simulink model "QR2Dsim"  (R2013b)
settings: Solver=ode3  StartTime=0.0  StopTime=Tend_sim  FixedStep=.01  RelTol=1e-3
values from neighbouring files (symbols this model uses):
  b = 0.1    [QR2Drunfile.m]
  ctauf = 8.004e-3    (= 0.008004)    [QR2Drunfile.m]
  d = 0.1    [QR2Drunfile.m]
  DeltaR = [0.2; -0.1; 0.02]    [QR2Drunfile.m]
  Deltax = [-0.5; 0.2; 1]    [QR2Drunfile.m]
  dxL0 = 0    [QR2Drunfile.m]
  dyL0 = 0    [QR2Drunfile.m]
  dzL0 = 0    [QR2Drunfile.m]
  e3 = [0;0;1]    [QR2Drunfile.m]
  fc = (mQ+mL)*g    (= 44.5374)    [QR2Drunfile.m]
  fsat = [-1000 1000]    [QR2Drunfile.m]
  g = 9.81    [QR2Drunfile.m]
  I = diag([Ixx Iyy Izz])    [QR2Drunfile.m]
  Ir = 0.5    [QR2Drunfile.m]
  Ixx = 0.0820    (= 0.082)    [QR2Drunfile.m]
  Iyy = 0    [QR2Drunfile.m]
  Izz = 0    [QR2Drunfile.m]
  kdL = 1.4    [QR2Drunfile.m]
  kdQ = 5.6*mQ*.75    (= 18.228)    [QR2Drunfile.m]
  kdxL = 1    [QR2Drunfile.m]
  kOmega = kOmega_phi*eye(3)    [QR2Drunfile.m]
  kpL = 1.2    [QR2Drunfile.m]
  kpQ = 16*mQ    (= 69.44)    [QR2Drunfile.m]
  kpxL = 5    [QR2Drunfile.m]
  kR = kR_phi*eye(3)    [QR2Drunfile.m]
  l = 0.315    [QR2Drunfile.m]
  lL = 0.4    [QR2Drunfile.m]
  mL = 0.2    [QR2Drunfile.m]
  mode = 2    [QR2Drunfile.m]
  mQ = 4.34    [QR2Drunfile.m]
  omega0 = [0;0;0]    [QR2Drunfile.m]
  phiL0 = deg2rad(190)    [QR2Drunfile.m]
  phiLd = 0    [QR2Drunfile.m]
  phiQ0 = deg2rad(0)    [QR2Drunfile.m]
  phiQd = 0    [QR2Drunfile.m]
  pL0 = 0    [QR2Drunfile.m]
  pQ0 = 0    [QR2Drunfile.m]
  psiL0 = 0    [QR2Drunfile.m]
  psiQ0 = 0    [QR2Drunfile.m]
  qL0 = 0    [QR2Drunfile.m]
  qQ0 = 0    [QR2Drunfile.m]
  qvec0 = [0; sin(phiL0); cos(phiL0)]    [QR2Drunfile.m]
  Rinit = Rx    [QR2Drunfile.m]
  rL0 = 0    [QR2Drunfile.m]
  rQ0 = 0    [QR2Drunfile.m]
  thetaL0 = 0    [QR2Drunfile.m]
  thetaQ0 = 0    [QR2Drunfile.m]
  xLd = [0; 0; 0]    [QR2Drunfile.m]
undefined symbols (not defined in the file or in its folder): dx0, dy0, dz0, kv, kx, m, p0, q0, r0, x0, y0, z0
libraries: simulink_extras x10, vrlib x9, dspmathops x2
(part 2 of 2)

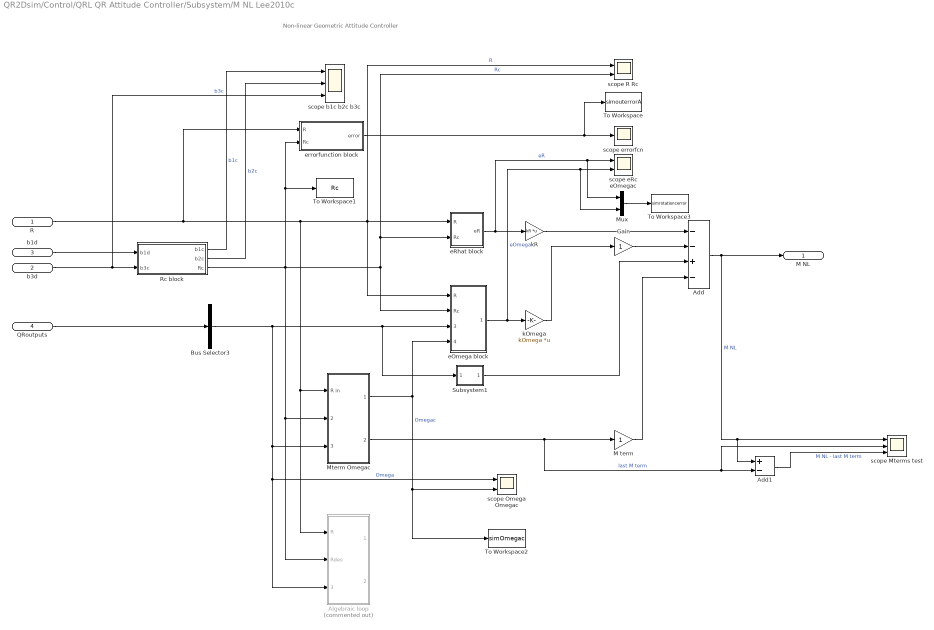
== system QR2Dsim/Control/QRL QR Attitude Controller/Subsystem/M NL Lee2010c ==
  note: Non-linear Geometric Attitude Controller
  R : Inport
  b3d : Inport  Port=2
  b1d : Inport  Port=3
  QRoutputs : Inport  Port=4
  Add : Sum  Inputs=--+-
  Add1 : Sum  Inputs=+-
  Algebraic loop : Subsystem  Commented=on
  Bus Selector3 : BusSelector  OutputSignals=OmegaL  OutputAsBus=on
  Gain : Gain
  M term : Gain
  Mterm Omegac : Subsystem
  Mux : Mux  Inputs=2
  Rc block : MATLAB Function  TreatAsAtomicUnit=on
  Subsystem1 : Subsystem
      mask Display: disp('\Omega \times I\Omega','texmode','on')
  To Workspace : ToWorkspace  VariableName=simouterrorA  SampleTime=-1  SaveFormat=Structure With Time
  To Workspace1 : ToWorkspace  VariableName=Rc  SampleTime=-1  SaveFormat=Structure With Time
  To Workspace2 : ToWorkspace  VariableName=simOmegac  SampleTime=-1  SaveFormat=Structure With Time
  To Workspace3 : ToWorkspace  VariableName=simrotationcerror  SampleTime=-1  SaveFormat=Structure With Time
  eOmega block : MATLAB Function  TreatAsAtomicUnit=on
  eRhat block : MATLAB Function  TreatAsAtomicUnit=on
  errorfunction block : MATLAB Function  TreatAsAtomicUnit=on
  kOmega : Gain  Gain=kOmega  Multiplication=Matrix(K*u)
  kR : Gain  Gain=kR  Multiplication=Matrix(K*u)
  scope Mterms test : Scope  NumInputPorts=3
      settings: YMin=-5~-5~-5  YMax=5~5~5  SaveName=ScopeData13
  scope Omega Omegac : Scope  NumInputPorts=2
      settings: ShowLegends=on  YMin=-5~-5  YMax=5~5  SaveName=scopeOmegac
  scope R Rc : Scope  NumInputPorts=2
      settings: ShowLegends=on  YMin=-5~-5  YMax=5~5  SaveName=ScopeData11
  scope b1c b2c b3c : Scope  NumInputPorts=3
      settings: ShowLegends=on  YMin=-5~-5~-5  YMax=5~5~5  SaveName=ScopeData10
  scope eRc eOmegac : Scope  NumInputPorts=2
      settings: YMin=-5~-5  YMax=5~5  SaveName=ScopeData8
  scope errorfcn : Scope
      settings: SaveName=scopeerrorfnc
  M NL : Outport
  wires:
  R/1 -> eOmega block/1(R), scope R Rc/1, eRhat block/1(R), Algebraic loop/1(R), Mterm Omegac/1(R in), errorfunction block/1(R)  "R"
  kR/1 -> Add/1
  kOmega/1 -> Gain/1
  QRoutputs/1 -> Bus Selector3/1
  Bus Selector3/1 -> eOmega block/3(Omega), Subsystem1/1(Omega), Algebraic loop/3(Omega), scope Omega Omegac/1, Mterm Omegac/3(Omega in)  "Omega"
  Rc block/3(Rc) -> errorfunction block/2(Rc), To Workspace1/1, eOmega block/2(Rc), scope R Rc/2, eRhat block/2(Rc), Algebraic loop/2(Rdes), Mterm Omegac/2(Rdes in)  "Rc"
  Subsystem1/1(Out1) -> Add/3
  Add/1 -> Add1/1, scope Mterms test/1, M NL/1  "M NL"
  errorfunction block/1(error) -> To Workspace/1, scope errorfcn/1
  Mterm Omegac/2(M term) -> M term/1, scope Mterms test/2, Add1/2  "last M term"
  Mterm Omegac/1(Omegades) -> To Workspace2/1, scope Omega Omegac/2, eOmega block/4(Omegac)  "Omegac"
  Gain/1 -> Add/2
  M term/1 -> Add/4
  Add1/1 -> scope Mterms test/3  "M NL - last M term"
  b3d/1 -> scope b1c b2c b3c/3, Rc block/2(b3c)  "b3c"
  b1d/1 -> Rc block/1(b1d)
  Rc block/2(b2c) -> scope b1c b2c b3c/2  "b2c"
  Rc block/1(b1c) -> scope b1c b2c b3c/1  "b1c"
  eRhat block/1(eR) -> Mux/1, scope eRc eOmegac/1, kR/1  "eR"
  eOmega block/1(eOmega) -> Mux/2, scope eRc eOmegac/2, kOmega/1  "eOmega"
  Mux/1 -> To Workspace3/1

== system QR2Dsim/Control/QRL QR Attitude Controller/Subsystem/M lin ==
  note: Linear Attitude Controller
  QRoutputs : Inport
  Add : Sum  Inputs=--
  Bus Selector3 : BusSelector  OutputSignals=OmegaL
  Constant : Constant  Value=[0;0;0]
  eR lin block : MATLAB Function  TreatAsAtomicUnit=on
  kOmega : Gain  Gain=kOmega  Multiplication=Matrix(K*u)
  kR : Gain  Gain=kR  Multiplication=Matrix(K*u)
  M lin : Outport
  wires:
  QRoutputs/1 -> Bus Selector3/1
  Bus Selector3/1 -> kOmega/1  "<OmegaL>"
  eR lin block/1(eRlin) -> kR/1  "eR lin"
  kR/1 -> Add/1
  kOmega/1 -> Add/2
  Add/1 -> M lin/1  "M lin"
  Constant/1 -> eR lin block/2(angles), eR lin block/1(anglesdes)  "anglesdes"

== system QR2Dsim/Control/QRL QR Attitude Controller/Subsystem1/Mterm Omegad ==
  R in : Inport
  Rdes in : Inport  Port=2
  Omega in : Inport  Port=3
  Derivative : Derivative  CoefficientInTFapproximation=c_der
  Gain : Gain
  Gain1 : Gain
  I : Gain  Gain=I  Multiplication=Matrix(K*u)
  Omegac block : MATLAB Function  TreatAsAtomicUnit=on
  Subsystem : Subsystem
  Sum : Sum  Inputs=|+-
  scope Omega Omegad : Scope  NumInputPorts=2
      settings: ShowLegends=on  YMin=-5~-5  YMax=5~5  SaveName=ScopeData22
  Omegades : Outport
  M term : Outport  Port=2
  wires:
  Omegac block/1(Omegad) -> scope Omega Omegad/2, Omegades/1, Subsystem/4(Omegad)  "Omegad"
  Rdes in/1 -> Derivative/1, Omegac block/1(Rd), Subsystem/2(Rd)
  R in/1 -> Subsystem/1(R)
  Omega in/1 -> scope Omega Omegad/1, Subsystem/3(Omega)
  Subsystem/1(Out1) -> Gain1/1
  Sum/1 -> I/1
  Gain/1 -> Sum/2
  Subsystem/2(Out2) -> Gain/1
  I/1 -> M term/1  "M term"
  Gain1/1 -> Sum/1
  Derivative/1 -> Omegac block/2(dRd)  "dRdesTR"

== system QR2Dsim/Control/QRL QR Attitude Controller/Subsystem1/Subsystem1 ==
  Omega : Inport
  Cross Product : vrlib/Utilities/Cross Product
  I : Gain  Gain=I  Multiplication=Matrix(K*u)
  Product1 : Product  Multiplication=Matrix(*)
  Terminator : Terminator
  fcnhat : MATLAB Function  TreatAsAtomicUnit=on
  Out1 : Outport
  wires:
  Omega/1 -> Cross Product/1, I/1, fcnhat/1(A)
  fcnhat/1(fcnhat) -> Product1/1
  I/1 -> Cross Product/2, Product1/2
  Cross Product/1 -> Out1/1
  Product1/1 -> Terminator/1

== system QR2Dsim/Control/QRL QR Attitude Controller/Subsystem/M NL Lee2010/Mterm Omegad ==
  R in : Inport
  Rdes in : Inport  Port=2
  Omega in : Inport  Port=3
  Derivative : Derivative  CoefficientInTFapproximation=c_der
  Gain : Gain
  Gain1 : Gain
  I : Gain  Gain=I  Multiplication=Matrix(K*u)
  Omegac block : MATLAB Function  TreatAsAtomicUnit=on
  Subsystem : Subsystem
  Sum : Sum  Inputs=|+-
  scope Omega Omegad : Scope  NumInputPorts=2
      settings: ShowLegends=on  YMin=-5~-5  YMax=5~5  SaveName=ScopeData22
  Omegades : Outport
  M term : Outport  Port=2
  wires:
  Omegac block/1(Omegad) -> scope Omega Omegad/2, Omegades/1, Subsystem/4(Omegad)  "Omegad"
  Rdes in/1 -> Derivative/1, Omegac block/1(Rd), Subsystem/2(Rd)
  R in/1 -> Subsystem/1(R)
  Omega in/1 -> scope Omega Omegad/1, Subsystem/3(Omega)
  Subsystem/1(Out1) -> Gain1/1
  Sum/1 -> I/1
  Gain/1 -> Sum/2
  Subsystem/2(Out2) -> Gain/1
  I/1 -> M term/1  "M term"
  Gain1/1 -> Sum/1
  Derivative/1 -> Omegac block/2(dRd)  "dRdesTR"

== system QR2Dsim/Control/QRL QR Attitude Controller/Subsystem/M NL Lee2010/Subsystem1 ==
  Omega : Inport
  Cross Product : vrlib/Utilities/Cross Product
  I : Gain  Gain=I  Multiplication=Matrix(K*u)
  Product1 : Product  Multiplication=Matrix(*)
  Terminator : Terminator
  fcnhat : MATLAB Function  TreatAsAtomicUnit=on
  Out1 : Outport
  wires:
  Omega/1 -> Cross Product/1, I/1, fcnhat/1(A)
  fcnhat/1(fcnhat) -> Product1/1
  I/1 -> Cross Product/2, Product1/2
  Cross Product/1 -> Out1/1
  Product1/1 -> Terminator/1

== system QR2Dsim/Control/QRL QR Attitude Controller/Subsystem/M NL Lee2010c/Algebraic loop ==
  R : Inport
  Rdes : Inport  Port=2
  Omega : Inport  Port=3
  Derivative1 : Derivative
  I : Gain  Gain=I  Multiplication=Matrix(K*u)
  I1 : Gain
  M term block : MATLAB Function  TreatAsAtomicUnit=on
  R block : Subsystem
      mask Display: disp('R_{d}^TR\prime_{d} = \Omega_{d,\times}','texmode','on')
  Scope Omegades : Scope  NumInputPorts=2
      settings: ShowLegends=on  YMin=-5~-5  YMax=5~5
  Scope fcnhat : Scope  NumInputPorts=2
      settings: ShowLegends=on  YMin=-5~-5  YMax=5~5  SaveName=ScopeData2
  Sum : Sum  Inputs=|+-
  M term : Outport
  Omegades : Outport  Port=2
  wires:
  Omega/1 -> M term block/3(Omega), Scope fcnhat/1  "Omega"
  Derivative1/1 -> Scope Omegades/2, M term block/5(dOmegades)  "dOmegades"
  I/1 -> M term/1
  R block/1(Omegades) -> Derivative1/1, Omegades/1, Scope fcnhat/2, Scope Omegades/1, M term block/4(Omegades)  "Omegades"
  R/1 -> M term block/1(R)
  Rdes/1 -> M term block/2(Rdes), R block/1(Rdes in)
  M term block/1(Out1) -> Sum/1
  M term block/2(Out2) -> I1/1
  Sum/1 -> I/1
  I1/1 -> Sum/2

== system QR2Dsim/Control/QRL QR Attitude Controller/Subsystem/M NL Lee2010c/Mterm Omegac ==
  R in : Inport
  Rdes in : Inport  Port=2
  Omega in : Inport  Port=3
  Derivative : Derivative  CoefficientInTFapproximation=c_der
  Gain : Gain
  Gain1 : Gain
  I : Gain  Gain=I  Multiplication=Matrix(K*u)
  Omegac block : MATLAB Function  TreatAsAtomicUnit=on
  Subsystem : Subsystem
  Sum : Sum  Inputs=|+-
  scope Omega Omegac : Scope  NumInputPorts=2
      settings: ShowLegends=on  YMin=-5~-5  YMax=5~5  SaveName=ScopeData22
  Omegades : Outport
  M term : Outport  Port=2
  wires:
  Rdes in/1 -> Subsystem/2(Rc), Omegac block/1(Rc), Derivative/1  "Rc"
  R in/1 -> Subsystem/1(R)  "R"
  Omega in/1 -> scope Omega Omegac/1, Subsystem/3(Omega)  "Omega"
  Subsystem/1(Out1) -> Gain1/1
  Sum/1 -> I/1
  Gain/1 -> Sum/2
  Subsystem/2(Out2) -> Gain/1
  I/1 -> M term/1  "M term"
  Gain1/1 -> Sum/1
  Omegac block/1(Omegac) -> Subsystem/4(Omegac), scope Omega Omegac/2, Omegades/1  "Omegac"
  Derivative/1 -> Omegac block/2(dRc)  "dRc"

== system QR2Dsim/Control/QRL QR Attitude Controller/Subsystem/M NL Lee2010c/Subsystem1 ==
  Omega : Inport
  Cross Product : vrlib/Utilities/Cross Product
  I : Gain  Gain=I  Multiplication=Matrix(K*u)
  Product1 : Product  Multiplication=Matrix(*)
  Terminator : Terminator
  fcnhat : MATLAB Function  TreatAsAtomicUnit=on
  Out1 : Outport
  wires:
  Omega/1 -> Cross Product/1, I/1, fcnhat/1(A)
  fcnhat/1(fcnhat) -> Product1/1
  I/1 -> Cross Product/2, Product1/2
  Cross Product/1 -> Out1/1
  Product1/1 -> Terminator/1

== system QR2Dsim/Control/QRL QR Attitude Controller/Subsystem1/Mterm Omegad/Subsystem ==
  R : Inport
  Rd : Inport  Port=2
  Omega : Inport  Port=3
  Omegad : Inport  Port=4
  Derivative1 : Derivative
  M term block : MATLAB Function  TreatAsAtomicUnit=on
  Scope Mterms : Scope  NumInputPorts=2
      settings: ShowLegends=on  YMin=-5~-5  YMax=5~5  SaveName=ScopeData23
  Scope Omega Omegad : Scope  NumInputPorts=2
      settings: ShowLegends=on  YMin=-5~-5  YMax=5~5  SaveName=ScopeData2
  Scope Omegad dOmegad : Scope  NumInputPorts=2
      settings: ShowLegends=on  YMin=-5~-5  YMax=5~5
  Scope R Rd : Scope  NumInputPorts=3
      settings: ShowLegends=on  YMin=-5~-5~-5  YMax=5~5~5  SaveName=ScopeData24
  Out1 : Outport
  Out2 : Outport  Port=2
  wires:
  Omega/1 -> M term block/3(Omega), Scope Omega Omegad/1  "Omega"
  Derivative1/1 -> Scope Omegad dOmegad/2, M term block/5(dOmegad)  "dOmegad"
  M term block/1(Out1) -> Scope Mterms/1, Out1/1
  Omegad/1 -> Derivative1/1, Scope Omega Omegad/2, Scope Omegad dOmegad/1, M term block/4(Omegad)  "Omegad"
  R/1 -> Scope R Rd/1, M term block/1(R)
  Rd/1 -> Scope R Rd/2, M term block/2(Rd)  "Rd"
  M term block/2(Out2) -> Scope Mterms/2, Out2/1
  M term block/3(Out3) -> Scope R Rd/3

== system QR2Dsim/Control/QRL QR Attitude Controller/Subsystem/M NL Lee2010/Mterm Omegad/Subsystem ==
  R : Inport
  Rd : Inport  Port=2
  Omega : Inport  Port=3
  Omegad : Inport  Port=4
  Derivative1 : Derivative
  M term block : MATLAB Function  TreatAsAtomicUnit=on
  Scope Mterms : Scope  NumInputPorts=2
      settings: ShowLegends=on  YMin=-5~-5  YMax=5~5  SaveName=ScopeData23
  Scope Omega Omegad : Scope  NumInputPorts=2
      settings: ShowLegends=on  YMin=-5~-5  YMax=5~5  SaveName=ScopeData2
  Scope Omegad dOmegad : Scope  NumInputPorts=2
      settings: ShowLegends=on  YMin=-5~-5  YMax=5~5
  Scope R Rd : Scope  NumInputPorts=3
      settings: ShowLegends=on  YMin=-5~-5~-5  YMax=5~5~5  SaveName=ScopeData24
  Out1 : Outport
  Out2 : Outport  Port=2
  wires:
  Omega/1 -> M term block/3(Omega), Scope Omega Omegad/1  "Omega"
  Derivative1/1 -> Scope Omegad dOmegad/2, M term block/5(dOmegad)  "dOmegad"
  M term block/1(Out1) -> Scope Mterms/1, Out1/1
  Omegad/1 -> Derivative1/1, Scope Omega Omegad/2, Scope Omegad dOmegad/1, M term block/4(Omegad)  "Omegad"
  R/1 -> Scope R Rd/1, M term block/1(R)
  Rd/1 -> Scope R Rd/2, M term block/2(Rd)  "Rd"
  M term block/2(Out2) -> Scope Mterms/2, Out2/1
  M term block/3(Out3) -> Scope R Rd/3

== system QR2Dsim/Control/QRL QR Attitude Controller/Subsystem/M NL Lee2010c/Algebraic loop/R block ==
  Rdes in : Inport
  Integrator : Integrator  InitialConditionSource=external  ContinuousStateAttributes='R'
  Math Function : Math  Operator=transpose  SaturateOnIntegerOverflow=on
  Product : Product  Inputs=**  Multiplication=Matrix(*)
  Product1 : Product  Inputs=**  Multiplication=Matrix(*)
  v block : MATLAB Function  TreatAsAtomicUnit=on
  Omegades : Outport
  wires:
  Rdes in/1 -> Integrator/2
  Integrator/1 -> Product/1, Math Function/1
  Math Function/1 -> Product1/1
  Product/1 -> Product1/2, Integrator/1
  Product1/1 -> v block/1(hat), Product/2
  v block/1(vec) -> Omegades/1

== system QR2Dsim/Control/QRL QR Attitude Controller/Subsystem/M NL Lee2010c/Mterm Omegac/Subsystem ==
  R : Inport
  Rc : Inport  Port=2
  Omega : Inport  Port=3
  Omegac : Inport  Port=4
  Derivative1 : Derivative
  M term block : MATLAB Function  TreatAsAtomicUnit=on
  Scope Mterms : Scope  NumInputPorts=2
      settings: ShowLegends=on  YMin=-5~-5  YMax=5~5  SaveName=ScopeData23
  Scope Omega Omegac : Scope  NumInputPorts=2
      settings: ShowLegends=on  YMin=-5~-5  YMax=5~5  SaveName=ScopeData2
  Scope Omegac dOmegac : Scope  NumInputPorts=2
      settings: ShowLegends=on  YMin=-5~-5  YMax=5~5
  Scope R Rdes : Scope  NumInputPorts=3
      settings: ShowLegends=on  YMin=-5~-5~-5  YMax=5~5~5  SaveName=ScopeData24
  Out1 : Outport
  Out2 : Outport  Port=2
  wires:
  Omega/1 -> M term block/3(Omega), Scope Omega Omegac/1  "Omega"
  Derivative1/1 -> Scope Omegac dOmegac/2, M term block/5(dOmegac)  "dOmegac"
  M term block/1(Out1) -> Scope Mterms/1, Out1/1
  Omegac/1 -> Derivative1/1, Scope Omega Omegac/2, Scope Omegac dOmegac/1, M term block/4(Omegac)  "Omegac"
  R/1 -> Scope R Rdes/1, M term block/1(R)  "R"
  Rc/1 -> Scope R Rdes/2, M term block/2(Rc)  "Rc"
  M term block/2(Out2) -> Out2/1, Scope Mterms/2
  M term block/3(Out3) -> Scope R Rdes/3

== matlab function QR2Dsim/QR Subsystem/omegarot block/fcnomega ==
  data: var input; M input size=3; f input; omegai output size=4
function omegai = fcn(var,M,f)
%omega = [omega_1^2;omega_2^2;omega_3^2;omega_4^2]

b = var(1);
d = var(2);
l = var(3);

%check if Gamma is invertible?
Gamma = [b b b b;0 -l*b 0 l*b;l*b 0 -l*b 0;-d d -d d];

QRinput = [f;M];

omegai = Gamma\QRinput;

== matlab function QR2Dsim/QR Subsystem/fi block/fcnf ==
  data: var input; M input size=3; f input; fi output size=4
function fi = fcn(var,M, f)
%omega = [omega_1^2;omega_2^2;omega_3^2;omega_4^2]

l = var(1);
ctauf = var(2);

%check if Gamma is invertible?
Gamma = [1 1 1 1;0 -l 0 l;l 0 -l 0;-ctauf ctauf -ctauf ctauf];

QRinput = [f;M];

fi = Gamma\QRinput;

== matlab function QR2Dsim/QR Subsystem/R block/MATLAB Function1 ==
  data: R input size=[3 3]; RR output size=[3 3]
function RR = fcn(R)
%#codegen
RR = R*R.';

== matlab function QR2Dsim/QR Subsystem/dOmega block/Subsystem2/fcnhat1 ==
  data: A input; fcnhat output
function fcnhat = fcn(A)

a = A(1);
b = A(2);
c = A(3);
fcnhat = [0 -c b; 
          c 0 -a;
         -b a 0];

== matlab function QR2Dsim/Control/QRL QR Attitude Controller/Subsystem1/Mterm Omegad/Omegac block ==
  data: Rd input size=[3 3]; dRd input size=[3 3]; Omegad output size=3
function Omegad = fcnOmegad(Rd,dRd)

Omegadhat = Rd.'*dRd;
Omegad = [Omegadhat(6);-Omegadhat(3);Omegadhat(2)];

== matlab function QR2Dsim/QR Subsystem/dOmega block/Subsystem2/fcnomega ==
  data: omega input; fcnomega output
function fcnomega = fcn(omega)

fcnomega = omega(2)+omega(4)-omega(1)-omega(3);

== matlab function QR2Dsim/QR-Load Subsystem/R block/dR block ==
  data: R input size=[3 3]; dR output size=[3 3]; Omega input size=3
function dR = fcn(R,Omega)
%#codegen
p = Omega(1);
q = Omega(2);
r = Omega(3);

Omegahat = [0 -r  q;
            r  0 -p;
           -q  p  0];

dR = R*Omegahat;
% R1 = R;

== matlab function QR2Dsim/Control/QRL QR Attitude Controller/Subsystem/M NL Lee2010/eRhat block ==
  data: R input size=[3 3]; Rdes input size=[3 3]; eR output size=3
function eR = fcnR(R,Rdes)
% Z-X-Y psi-phi-theta

eRhat = (Rdes.'*R-R.'*Rdes);

eR = 0.5*[eRhat(6);-eRhat(3);eRhat(2)];

== matlab function QR2Dsim/QR-Load Subsystem/dOmegaQ block/Subsystem1/fcnhat ==
  data: A input size=[3 1]; fcnhat output size=[3 3]
function fcnhat = fcn(A)

a = A(1);
b = A(2);
c = A(3);
fcnhat = [0 -c b; 
          c 0 -a;
         -b a 0];

== matlab function QR2Dsim/Control/QRL QR Attitude Controller/Subsystem/M lin/eR lin block ==
  data: anglesdes input size=[3 1]; angles input size=[3 1]; eRlin output size=3
function eRlin = fcnR(anglesdes,angles)
% Z-X-Y psi-phi-theta
% Rdes =  R(psi0+dpsi, dphi, dtheta)
% R = R(psi0,0,0)

% dphi   = anglesdes(1) - angles(1);
% dtheta = anglesdes(2) - angles(2);
% dpsi   = anglesdes(3) - angles(3);

dphi   = angles(1);
dtheta = angles(2);
dpsi   = angles(3);

eRlin  = [dphi; dtheta; dpsi];
% Of toch: 
% eRlin  = [-dphi; -dtheta; -dpsi];

== matlab function QR2Dsim/Control/QRL QR Attitude Controller/Subsystem/M NL Lee2010/eOmega block ==
  data: R input size=[3 3]; Rd input size=[3 3]; eOmega output size=3; Omega input size=[3 1]; Omegad input size=[3 1]
function eOmega = fcnR(R,Rd,Omega,Omegad)
% Z-X-Y psi-phi-theta

eOmega = Omega - R.'*Rd*Omegad;

== matlab function QR2Dsim/Control/QRL QR Attitude Controller/Subsystem/M NL Lee2010/Rdes block ==
  data: b2d output; b1d input size=[3 1]; Rdes output size=[3 3]; b3d input size=[3 1]
function [b2d,Rdes] = fcnRdes(b1d,b3d)
%
b2d = cross(b3d,b1d);
Rdes = [b1d b2d b3d];

== matlab function QR2Dsim/QR-Load Subsystem/dOmegaQ block/Subsystem2/fcnhat1 ==
  data: A input; fcnhat output
function fcnhat = fcn(A)

a = A(1);
b = A(2);
c = A(3);
fcnhat = [0 -c b; 
          c 0 -a;
         -b a 0];

== matlab function QR2Dsim/Control/QRL QR Attitude Controller/Subsystem/M NL Lee2010/Subsystem1/fcnhat ==
  data: A input size=[3 1]; fcnhat output size=[3 3]
function fcnhat = fcn(A)

a = A(1);
b = A(2);
c = A(3);
fcnhat = [0 -c b; 
          c 0 -a;
         -b a 0];

== matlab function QR2Dsim/QR-Load Subsystem/dOmegaQ block/Subsystem2/fcnomega ==
  data: omega input; fcnomega output
function fcnomega = fcn(omega)

fcnomega = omega(2)+omega(4)-omega(1)-omega(3);

== matlab function QR2Dsim/QR Subsystem/R block/dR block ==
  data: R input size=[3 3]; dR output size=[3 3]; Omega input size=3
function dR = fcn(R,Omega)
%#codegen
p = Omega(1);
q = Omega(2);
r = Omega(3);

Omegahat = [0 -r  q;
            r  0 -p;
           -q  p  0];

dR = R*Omegahat;
% R1 = R;

== matlab function QR2Dsim/Control/QRL QR Attitude Controller/Subsystem/M NL Lee2010/errorfunction block ==
  data: R input size=[3 3]; Rdes input size=[3 3]; error output
function error = fcn(R,Rdes)

error = 0.5*trace(eye(3)-Rdes.'*R);

== matlab function QR2Dsim/QR Subsystem/dOmega block/Subsystem1/fcnhat ==
  data: A input size=[3 1]; fcnhat output size=[3 3]
function fcnhat = fcn(A)

a = A(1);
b = A(2);
c = A(3);
fcnhat = [0 -c b; 
          c 0 -a;
         -b a 0];

== matlab function QR2Dsim/Control/QRL QR Attitude Controller/Subsystem/M NL Lee2010c/Algebraic loop/M term block ==
  data: R input size=[3 3]; Rdes input size=[3 3]; Out1 output size=3; Omega input size=3; Omegades input size=3; dOmegades input; Out2 output
function [Out1,Out2] = fcnR(R,Rdes,Omega,Omegades,dOmegades)
% Z-X-Y psi-phi-theta

p = Omega(1);
q = Omega(2);
r = Omega(3);

Omegahat = [0 -r  q;
            r  0 -p;
           -q  p  0];

Out1 = Omegahat*R.'*Rdes*Omegades;
Out2 = R.'*Rdes*dOmegades;

== matlab function QR2Dsim/Control/QRL QR Attitude Controller/Subsystem/M NL Lee2010/Mterm Omegad/Subsystem/M term block ==
  data: R input size=[3 3]; Rd input size=[3 3]; Out1 output size=3; Omega input size=3; Omegad input size=3; dOmegad input; Out2 output; Out3 output
function [Out1,Out2,Out3] = fcnR(R,Rd,Omega,Omegad,dOmegad)
% Z-X-Y psi-phi-theta

p = Omega(1);
q = Omega(2);
r = Omega(3);

Omegahat = [0 -r  q;
            r  0 -p;
           -q  p  0];

Out1 = Omegahat*R.'*Rd*Omegad;
Out2 = R.'*Rd*dOmegad;
Out3 = R.'*Rd;

== matlab function QR2Dsim/Control/QRL QR Attitude Controller/Subsystem/M NL Lee2010c/Algebraic loop/R block/v block ==
  data: hat input size=[3 3]; vec output size=3
function vec = fcn(hat)

vec = [hat(6); -hat(3); hat(2)];

== matlab function QR2Dsim/Control/QRL QR Attitude Controller/Subsystem/M NL Lee2010c/Rc block ==
  data: b1c output; b2c output; b1d input size=[3 1]; Rc output size=[3 3]; b3c input size=[3 1]
function [b1c,b2c,Rc] = fcnRc(b1d,b3c)
%
b1c = -cross(b3c,(cross(b3c,b1d)/norm(cross(b3c,b1d))));
% b1c = -cross(b3c,normc(cross(b3c,b1d)));
b2c = cross(b3c,b1c);
Rc = [b1c b2c b3c];
% Rc = Rc.';

== matlab function QR2Dsim/Control/QRL QR Attitude Controller/Subsystem/M NL Lee2010c/Mterm Omegac/Omegac block ==
  data: Rc input size=[3 3]; dRc input size=[3 3]; Omegac output size=3
function Omegac = fcnOmegac(Rc,dRc)

Omegachat = Rc.'*dRc;
Omegac = [Omegachat(6);-Omegachat(3);Omegachat(2)];

== matlab function QR2Dsim/Control/QRL QR Attitude Controller/Subsystem/M NL Lee2010c/Mterm Omegac/Subsystem/M term block ==
  data: R input size=[3 3]; Rc input size=[3 3]; Out1 output size=3; Omega input size=3; Omegac input size=3; dOmegac input; Out2 output; Out3 output
function [Out1,Out2,Out3] = fcnMterm(R,Rc,Omega,Omegac,dOmegac)
% Z-X-Y psi-phi-theta

p = Omega(1);
q = Omega(2);
r = Omega(3);

Omegahat = [0 -r  q;
            r  0 -p;
           -q  p  0];

Out1 = Omegahat*R.'*Rc*Omegac;
Out2 = R.'*Rc*dOmegac;
Out3 = R.'*Rc;

== matlab function QR2Dsim/Control/QRL QR Attitude Controller/Subsystem/M NL Lee2010c/Subsystem1/fcnhat ==
  data: A input size=[3 1]; fcnhat output size=[3 3]
function fcnhat = fcn(A)

a = A(1);
b = A(2);
c = A(3);
fcnhat = [0 -c b; 
          c 0 -a;
         -b a 0];

== matlab function QR2Dsim/Control/QRL QR Attitude Controller/Subsystem/M NL Lee2010c/eOmega block ==
  data: R input size=[3 3]; Rc input size=[3 3]; eOmega output size=3; Omega input size=[3 1]; Omegac input size=[3 1]
function eOmega = fcneOmega(R,Rc,Omega,Omegac)
% Z-X-Y psi-phi-theta

eOmega = Omega - R.'*Rc*Omegac;

== matlab function QR2Dsim/Control/QRL QR Attitude Controller/Subsystem/M NL Lee2010c/eRhat block ==
  data: R input size=[3 3]; Rc input size=[3 3]; eR output size=3
function eR = fcneRc(R,Rc)
% Z-X-Y psi-phi-theta

eRhat = (Rc.'*R-R.'*Rc);
eR = 0.5*[eRhat(6);-eRhat(3);eRhat(2)];

== matlab function QR2Dsim/Control/QRL QR Attitude Controller/Subsystem/M NL Lee2010c/errorfunction block ==
  data: R input size=[3 3]; Rc input size=[3 3]; error output
function error = fcnerrorA(R,Rc)

error = 0.5*trace(eye(3)-Rc.'*R);

== matlab function QR2Dsim/Control/QRL QR Attitude Controller/Subsystem/M NL Lee2010/Mterm Omegad/Omegac block ==
  data: Rd input size=[3 3]; dRd input size=[3 3]; Omegad output size=3
function Omegad = fcnOmegad(Rd,dRd)

Omegadhat = Rd.'*dRd;
Omegad = [Omegadhat(6);-Omegadhat(3);Omegadhat(2)];

== matlab function QR2Dsim/QR-Load Subsystem/fi block/fcnf ==
  data: var input; M input size=3; f input; fi output size=4
function fi = fcn(var,M, f)
%omega = [omega_1^2;omega_2^2;omega_3^2;omega_4^2]

l = var(1);
ctauf = var(2);

%check if Gamma is invertible?
Gamma = [1 1 1 1;0 -l 0 l;l 0 -l 0;-ctauf ctauf -ctauf ctauf];

QRinput = [f;M];

fi = Gamma\QRinput;

== matlab function QR2Dsim/QR-Load Subsystem/omegarot block/fcnomega ==
  data: var input; M input size=3; f input; omegai output size=4
function omegai = fcn(var,M,f)
%omega = [omega_1^2;omega_2^2;omega_3^2;omega_4^2]

b = var(1);
d = var(2);
l = var(3);

%check if Gamma is invertible?
Gamma = [b b b b;0 -l*b 0 l*b;l*b 0 -l*b 0;-d d -d d];

QRinput = [f;M];

omegai = Gamma\QRinput;

== matlab function QR2Dsim/QR-Load Subsystem/dxL block ==
  data: varddxL input; dq input; ddxL output size=3; q input size=3; R input size=[3 3]; f input size=1
function ddxL = fcn(varddxL,dq,q,R,f)

mQ = varddxL(1);
g  = varddxL(2);
mL = varddxL(3);
lL = varddxL(4);

e3 = [0;0;1];



ddxL = ( ( (dot(q,(f*R*e3)) - mQ*lL*dot(dq,dq)) * q ) / (mQ+mL) ) - g*e3;

== matlab function QR2Dsim/Control/QRL QR Attitude Controller/Subsystem1/Mterm Omegad/Subsystem/M term block ==
  data: R input size=[3 3]; Rd input size=[3 3]; Out1 output size=3; Omega input size=3; Omegad input size=3; dOmegad input; Out2 output; Out3 output
function [Out1,Out2,Out3] = fcnR(R,Rd,Omega,Omegad,dOmegad)
% Z-X-Y psi-phi-theta

p = Omega(1);
q = Omega(2);
r = Omega(3);

Omegahat = [0 -r  q;
            r  0 -p;
           -q  p  0];

Out1 = Omegahat*R.'*Rd*Omegad;
Out2 = R.'*Rd*dOmegad;
Out3 = R.'*Rd;

== matlab function QR2Dsim/Control/QRL QR Attitude Controller/Subsystem1/Rdes block ==
  data: b2d output; b1d input size=[3 1]; Rdes output size=[3 3]; b3d input size=[3 1]
function [b2d,Rdes] = fcnRdes(b1d,b3d)
%
b2d = cross(b3d,b1d);
Rdes = [b1d b2d b3d];

== matlab function QR2Dsim/Control/QRL QR Attitude Controller/Subsystem1/Subsystem1/fcnhat ==
  data: A input size=[3 1]; fcnhat output size=[3 3]
function fcnhat = fcn(A)

a = A(1);
b = A(2);
c = A(3);
fcnhat = [0 -c b; 
          c 0 -a;
         -b a 0];

== matlab function QR2Dsim/Control/QRL QR Attitude Controller/Subsystem1/eOmega block ==
  data: R input size=[3 3]; Rd input size=[3 3]; eOmega output size=3; Omega input size=[3 1]; Omegad input size=[3 1]
function eOmega = fcnR(R,Rd,Omega,Omegad)
% Z-X-Y psi-phi-theta

eOmega = Omega - R.'*Rd*Omegad;

== matlab function QR2Dsim/Control/QRL QR Attitude Controller/Subsystem1/eRhat block ==
  data: R input size=[3 3]; Rdes input size=[3 3]; eR output size=3
function eR = fcnR(R,Rdes)
% Z-X-Y psi-phi-theta

eRhat = (Rdes.'*R-R.'*Rdes);

eR = 0.5*[eRhat(6);-eRhat(3);eRhat(2)];

== matlab function QR2Dsim/Control/QRL QR Attitude Controller/Subsystem1/errorfunction block ==
  data: R input size=[3 3]; Rdes input size=[3 3]; error output
function error = fcn(R,Rdes)

error = 0.5*trace(eye(3)-Rdes.'*R);

== matlab function QR2Dsim/QR-Load Subsystem/2D R block ==
  data: angleQ input; R output
function R = fcn(angleQ)

phiQ = angleQ(3);

R = [1 0          0;
     0 cos(phiQ) -sin(phiQ);
     0 sin(phiQ)  cos(phiQ)];
